simulink model "Copy_2_of_trial_with_intermediate_tanks"  (R2024b)
settings: Solver=ode15s  StartTime=0.0  StopTime=T_sim  FixedStep=1e-6  MaxStep=1e-6  RelTol=1e-6
InitFcn:
  | param = struct();
  | 
  | % Fluid properties
  | param.rho = 870;
  | 
  | % Pressure Rails
  | param.P_H = 7e6;
  | param.P_M = 3.5e6;
  | param.P_L = 101325;
  | 
  | % Linear Actuator Chamber
  | param.V1_0 = 100e-6;
  | param.Acap = pi*(0.5*2.54)^2*1e-4;
  | 
  | % Intermediary volumes
  | param.V3_0 = 25e-6;
  | param.V4_0 = 25e-6;
  | 
  | % Fluid
  | param.beta = 1.8e9;
  | param.air = 0.05;
  | 
  | % Valve
  | param.max_Avt = 0.5*0.25*pi*(20e-3)^2;
  | param.Cd = 0.6;
  | 
  | % Valve Dynamics
  | param.wn = 50*2*pi;
  | param.zeta = 1;
  | 
  | % Hydraulic Pump/Motor
  | param.J_hyd = 3000e-7;
  | param.D = 0.8e-6;    % In cc/rev
  | 
  | % Electric Motor/Generator
  | param.J_elec = 3060e-7;
  | param.Kt = 109e-3;
settings Model: Creator=ibrah408  LastModifiedBy=user
settings SolverCC: MaxConsecutiveZCs=10000
settings RTWCC: GPUComputeCapability=3.5

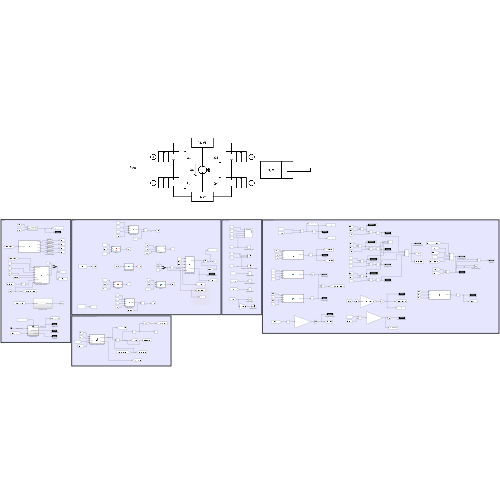
[thumbnail: Simulink's stored preview of the top-level diagram]
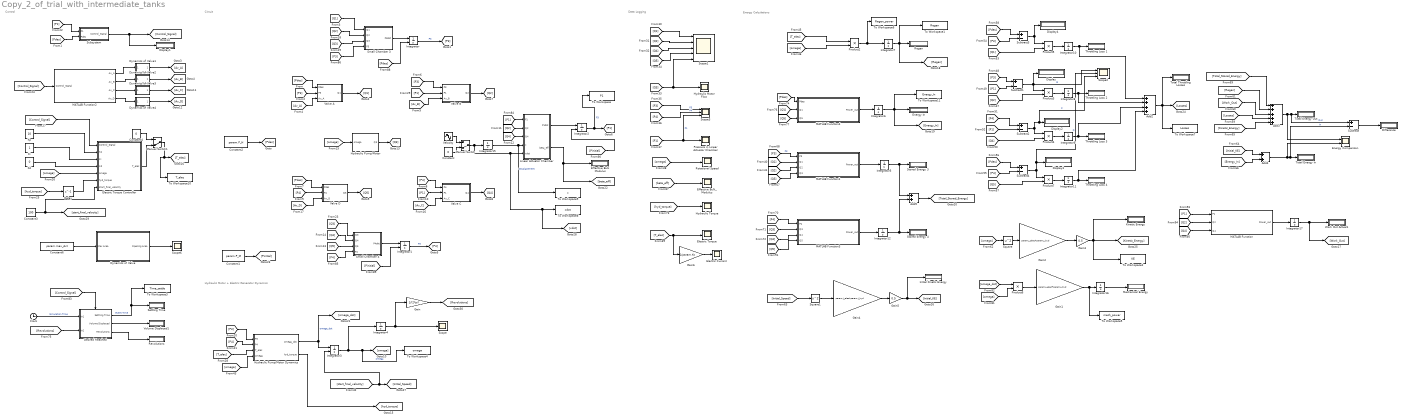
== system Copy_2_of_trial_with_intermediate_tanks ==
  note: Energy Calculations
  note: Data Logging
  note: Hydraulic Motor + Electric Generator Dynamics
  note: Circuit
  note: Control
  Add2 : Sum  Inputs=++++
  Add3 : Sum  Inputs=+++++
  Add4 : Sum
  Add5 : Sum
  Clock : Clock
  Constant : Constant  Value=0
  Constant1 : Constant  Value=param.P_M
  Constant2 : Constant  Value=param.P_H
  Constant3 : Constant  Value=100
  Constant4 : Constant  Value=0
  Constant6 : Constant  Value=param.max_Avt
  Delay : Delay  DelayLength=1
  Desired Reached : Subsystem  TreatAsAtomicUnit=on
  Difference : Display
  Display{,1..4} (5 alike) : Display
  Dynamics of Valve : Subsystem
  Dynamics of Valve1 : Subsystem
  Dynamics of Valve2 : Subsystem
  Dynamics of Valve3 : Subsystem
  Dynamics of Valve4 : Subsystem
  Effective Bulk Modulus : Display
  Effective Bulk_Modulus : Scope
  Electric Current : Scope
  Electric Torque : Scope
  Electric Torque Controller : MATLAB Function  TreatAsAtomicUnit=on
  Energy Comparison : Scope  NumInputPorts=2
  Energy In : Display
  Gain : Gain  Gain=1/(2*pi)
  Gain1 : Gain  Gain=param.J_elec+param.J_hyd
  Gain2 : Gain  Gain=param.J_elec+param.J_hyd
  Gain3 : Gain  Gain=0.5
  Gain4 : Gain  Gain=param.J_elec+param.J_hyd
  Gain5 : Gain  Gain=0.5
  Gain6 : Gain  Gain=1/param.Kt
  Hydraulic Motor Flow : Scope
  Hydraulic Pump/Motor : MATLAB Function  TreatAsAtomicUnit=on
  Hydraulic Pump/Motor Dynamics : MATLAB Function  TreatAsAtomicUnit=on
  Hydraulic Torque : Scope
  Initial Kinetic Energy : Display
  Integrator : Integrator  InitialConditionSource=external  InitialCondition=param.P_M
  Integrator1 : Integrator  InitialConditionSource=external  InitialCondition=param.P_M
  Integrator{4..12,15..17} (12 alike) : Integrator
  Integrator2 : Integrator  InitialConditionSource=external  InitialCondition=param.P_M
  Integrator3 : Integrator  InitialConditionSource=external
  Kd : Constant  Value=0
  Ki : Constant
  Kinetic Energy : Display
  Kp : Constant  Value=10
  Linear Actuator Chamber : MATLAB Function  TreatAsAtomicUnit=on
  MATLAB Function : MATLAB Function  TreatAsAtomicUnit=on
  MATLAB Function1 : MATLAB Function  TreatAsAtomicUnit=on
  MATLAB Function2 : MATLAB Function  TreatAsAtomicUnit=on
  MATLAB Function3 : MATLAB Function  TreatAsAtomicUnit=on
  MATLAB Function4 : MATLAB Function  TreatAsAtomicUnit=on
  Manual Switch : ManualSwitch  CurrentSetting=0
  Manual Switch1 : ManualSwitch  CurrentSetting=0
  Mechanical Energy : Display
  Pressure in Linear Actuator Chamber : Scope
  Product{2..7} (6 alike) : Product
  Regen : Display
  Revolutions : Display
  Rotational Speed : Scope
  Scope : Scope
  Scope1 : Scope  NumInputPorts=5
  Scope2 : Scope  NumInputPorts=3
  Scope3 : Scope  NumInputPorts=3
  Scope6 : Scope
  Settling Time : Display
  Small Chamber 3 : MATLAB Function  TreatAsAtomicUnit=on
  Small Chamber 4 : MATLAB Function  TreatAsAtomicUnit=on
  Square : Math  Operator=square
  Square1 : Math  Operator=square
  Stored Energy 3 : Display
  Stored Energy 4 : Display
  Subsystem : Subsystem
  Subtract{,1..4} (5 alike) : Sum  Inputs=+-
  Throttling Loss {1..4} (4 alike) : Display
  To Workspace : ToWorkspace  VariableName=P1  SaveFormat=Timeseries  SampleTime=-1
  To Workspace1 : ToWorkspace  VariableName=Regen  SaveFormat=Timeseries  SampleTime=-1
  To Workspace10 : ToWorkspace  VariableName=T_elec  SaveFormat=Timeseries  SampleTime=-1
  To Workspace11 : ToWorkspace  VariableName=Energy_In  SaveFormat=Timeseries  SampleTime=-1
  To Workspace2 : ToWorkspace  VariableName=KE  SaveFormat=Timeseries  SampleTime=-1
  To Workspace3 : ToWorkspace  VariableName=Time_settle  SaveFormat=Timeseries  SampleTime=-1
  To Workspace4 : ToWorkspace  VariableName=omega  SaveFormat=Timeseries  SampleTime=-1
  To Workspace5 : ToWorkspace  VariableName=mech_power  SaveFormat=Timeseries  SampleTime=-1
  To Workspace6 : ToWorkspace  VariableName=Regen_power  SaveFormat=Timeseries  SampleTime=-1
  To Workspace7 : ToWorkspace  VariableName=Losses  SaveFormat=Timeseries  SampleTime=-1
  To Workspace8 : ToWorkspace  VariableName=xdot  SaveFormat=Timeseries  SampleTime=-1
  To Workspace9 : ToWorkspace  VariableName=x  SaveFormat=Timeseries  SampleTime=-1
  Total Energy In : Display
  Total Energy Out : Display
  Total Throttling Losses : Display
  Valve A : MATLAB Function  TreatAsAtomicUnit=on
  Valve B : MATLAB Function  TreatAsAtomicUnit=on
  Valve C : MATLAB Function  TreatAsAtomicUnit=on
  Valve D : MATLAB Function  TreatAsAtomicUnit=on
  Velocity : Sin  Amplitude=1e-2  Frequency=(2*pi)/0.2  Phase=pi/2  SampleTime=0
  Volume Displaced1 : Display
  Work Out Actual1 : Display
  wires:
  [Pdes] -> Valve A/1(Pdes)
  Small Chamber 3/1(P3dot) -> Integrator/1
  [Pdes] -> Integrator/2
  Constant2/1 -> [Pdes]
  [Pdes] -> Subsystem/2(Pdes)
  Integrator/1 -> [P3]  "P3"
  [P3] -> Valve A/2(P3)
  Valve A/1(Q1) -> [Q1]
  [Q1] -> Small Chamber 3/1(Q1)
  [Av_A] -> Valve A/3(Av_A)
  [Av_B] -> Valve B/3(Av_B)
  [P3] -> Valve B/1(P3)
  [Pdes] -> Valve D/1(Pdes)
  Small Chamber 4/1(P4dot) -> Integrator1/1
  [Pinitial] -> Integrator1/2
  Integrator1/1 -> [P4]  "P3"
  [P4] -> Valve C/1(P4)
  [P4] -> Valve D/2(P4)
  Linear Actuator Chamber/1(P1dot) -> Integrator2/1
  [Pinitial] -> Integrator2/2
  Integrator2/1 -> To Workspace/1, [P1]  "P3"
  [P1] -> Valve C/2(P1)
  Valve B/1(Q2) -> [Q2]
  [Q2] -> Linear Actuator Chamber/2(Q2)
  Valve C/1(Q4) -> [Q4]
  [Q4] -> Linear Actuator Chamber/3(Q4)
  Valve D/1(Q5) -> [Q5]
  [Q5] -> Small Chamber 4/3(Q5)
  [Q4] -> Small Chamber 4/2(Q4)
  Hydraulic Pump/Motor Dynamics/1(omega_dot) -> [omega_dot], Integrator3/1  "omega_dot"
  Integrator3/1 -> Integrator4/1, To Workspace4/1, [omega]  "omega"
  [omega] -> Hydraulic Pump/Motor/1(omega)
  [Av_C] -> Valve C/3(Av_C)
  [Av_D] -> Valve D/3(Av_D)
  [Q2] -> Small Chamber 3/2(Q2)
  Hydraulic Pump/Motor/1(Q3) -> [Q3]
  [Q3] -> Small Chamber 3/3(Q3)
  [P3] -> Hydraulic Pump/Motor Dynamics/1(P3)
  [P4] -> Hydraulic Pump/Motor Dynamics/2(P4)
  [P1] -> Subsystem/1(P1)
  [Q3] -> Small Chamber 4/1(Q3)
  Subsystem/1(Control_Signal) -> [Control_Signal], Display1/1
  [Control_Signal] -> MATLAB Function2/1(Control_Signal)
  Integrator4/1 -> Scope/1, Gain/1
  Gain/1 -> [Revolutions]
  Hydraulic Pump/Motor Dynamics/2(hyd_torque) -> [hyd_torque]
  [hyd_torque] -> Delay/1
  Delay/1 -> Electric Torque Controller/6(hyd_torque)
  [omega] -> Electric Torque Controller/5(omega)
  [Control_Signal] -> Electric Torque Controller/1(Control_Signal)
  [P1] -> Valve B/2(P1)
  [Q1] -> Scope1/1
  [Q2] -> Scope1/2
  [Q4] -> Scope1/3
  [Q5] -> Scope1/4
  [Q3] -> Scope1/5, Hydraulic Motor Flow/1
  [P3] -> Scope3/1  "P3"
  [P4] -> Scope3/2  "P4"
  [P1] -> Scope3/3, Pressure in Linear Actuator Chamber/1  "P1"
  [omega] -> Rotational Speed/1
  Integrator6/1 -> To Workspace11/1, [Energy_In], Energy In/1
  [T_elec] -> Product2/1
  [omega] -> Product2/2
  Product2/1 -> To Workspace6/1, Integrator7/1
  Integrator7/1 -> To Workspace1/1, [Regen], Regen/1
  Constant6/1 -> Dynamics of Valve/1(Max Area)
  Dynamics of Valve/1(Opening Area) -> Scope6/1
  MATLAB Function2/1(Av_A) -> Dynamics of Valve1/1(Max Area)
  Dynamics of Valve1/1(Opening Area) -> [Av_A]
  MATLAB Function2/2(Av_B) -> Dynamics of Valve2/1(Max Area)
  Dynamics of Valve2/1(Opening Area) -> [Av_B]
  MATLAB Function2/3(Av_C) -> Dynamics of Valve3/1(Max Area)
  Dynamics of Valve3/1(Opening Area) -> [Av_C]
  MATLAB Function2/4(Av_D) -> Dynamics of Valve4/1(Max Area)
  Dynamics of Valve4/1(Opening Area) -> [Av_D]
  Product4/1 -> Integrator9/1
  [Q2] -> Product3/2
  [P4] -> Subtract2/1
  Integrator11/1 -> Add2/4, Throttling Loss 4/1
  [P4] -> Subtract4/2
  [Pdes] -> Subtract4/1
  [P1] -> Subtract2/2
  Product7/1 -> Integrator11/1
  Integrator9/1 -> Add2/3, Throttling Loss 3/1
  Subtract3/1 -> Display4/1, Product5/1
  Product3/1 -> Integrator8/1
  [Pdes] -> Subtract3/1
  Add2/1 -> Total Throttling Losses/1, To Workspace7/1, [Losses]
  Subtract1/1 -> Scope2/1, Product3/1, Display/1  "B"
  Product5/1 -> Integrator10/1
  [P3] -> Subtract1/1
  Integrator8/1 -> Add2/2, Throttling Loss 2/1
  [P1] -> Subtract1/2
  [Q5] -> Product7/2
  Integrator10/1 -> Add2/1, Throttling Loss 1/1
  [P3] -> Subtract3/2
  Subtract4/1 -> Product7/1, Scope2/2, Display3/1  "D"
  [Q4] -> Product4/2
  Subtract2/1 -> Product4/1, Scope2/3, Display2/1  "C"
  [Q1] -> Product5/2
  [Regen] -> Add3/2
  [Work_Out] -> Add3/3
  [Losses] -> Add3/4
  Gain3/1 -> To Workspace2/1, [Kinetic_Energy], Kinetic Energy/1
  [omega] -> Square/1
  Square/1 -> Gain2/1
  Gain2/1 -> Gain3/1
  [Initial_Speed] -> Square1/1
  Gain4/1 -> Gain5/1
  Square1/1 -> Gain4/1
  Gain5/1 -> Initial Kinetic Energy/1, [Initial_KE]
  [Kinetic_Energy] -> Add3/5
  [Initial_KE] -> Add4/1
  [Energy_In] -> Add4/2
  Add4/1 -> Energy Comparison/2, Subtract/2, Total Energy In/1  "In"
  Add3/1 -> Energy Comparison/1, Subtract/1, Total Energy Out/1  "Out"
  Add5/1 -> [Total_Stored_Energy]
  [Total_Stored_Energy] -> Add3/1
  Integrator15/1 -> To Workspace9/1, Linear Actuator Chamber/4(x)  "Displacement"
  Velocity/1 -> Manual Switch/1
  Manual Switch/1 -> Integrator15/1, [xdot], To Workspace8/1, Linear Actuator Chamber/5(xdot)
  Constant/1 -> Manual Switch/2
  Product6/1 -> Gain1/1
  [omega] -> Product6/2
  Integrator16/1 -> Mechanical Energy/1
  [omega_dot] -> Product6/1
  Gain1/1 -> To Workspace5/1, Integrator16/1
  [Control_Signal] -> Desired Reached/Trigger
  Clock/1 -> Desired Reached/1(In1)  "Simulation Time"
  Desired Reached/1(Settling Time) -> Settling Time/1, To Workspace3/1  "Event Time"
  Linear Actuator Chamber/2(beta_eff) -> [beta_eff], Effective Bulk Modulus/1
  [P1] -> Linear Actuator Chamber/1(P1)
  [P4] -> Small Chamber 4/4(P4)
  [P3] -> Small Chamber 3/4(P3)
  [beta_eff] -> Effective Bulk_Modulus/1
  Constant1/1 -> [Pinitial]
  [Q4] -> MATLAB Function/3(Q4)
  [Q2] -> MATLAB Function/2(Q2)
  [P1] -> MATLAB Function/1(P1)
  MATLAB Function/1(Power_out) -> Integrator17/1
  Integrator17/1 -> Work Out Actual1/1, [Work_Out]
  [Q1] -> MATLAB Function1/2(Q1)
  [Q2] -> MATLAB Function1/3(Q2)
  [Q3] -> MATLAB Function1/4(Q3)
  [P3] -> MATLAB Function1/1(P3)  "P3"
  MATLAB Function1/1(Power_out) -> Integrator5/1
  Integrator5/1 -> Add5/1, Stored Energy 3/1
  MATLAB Function3/1(Power_out) -> Integrator12/1
  Integrator12/1 -> Add5/2, Stored Energy 4/1
  [P4] -> MATLAB Function3/1(P4)
  [Q3] -> MATLAB Function3/2(Q3)
  [Q4] -> MATLAB Function3/3(Q4)
  [Q5] -> MATLAB Function3/4(Q5)
  Subtract/1 -> Difference/1
  [hyd_torque] -> Hydraulic Torque/1
  [Revolutions] -> Desired Reached/2(In2)
  Desired Reached/2(Volume Displaced) -> Volume Displaced1/1
  Desired Reached/3(Revolutions) -> Revolutions/1
  [Pdes] -> MATLAB Function4/1(Pdes)
  [Q1] -> MATLAB Function4/2(Q1)
  [Q5] -> MATLAB Function4/3(Q5)
  MATLAB Function4/1(Power_out) -> Integrator6/1
  [T_elec] -> Electric Torque/1, Gain6/1
  Gain6/1 -> Electric Current/1
  Constant3/1 -> Electric Torque Controller/7(start_final_velocity), [start_final_velocity]
  [start_final_velocity] -> [Initial_Speed], Integrator3/2
  [T_elec] -> Hydraulic Pump/Motor Dynamics/3(T_elec)
  Constant4/1 -> Manual Switch1/1
  Electric Torque Controller/1(T_elec) -> Manual Switch1/2
  Manual Switch1/1 -> To Workspace10/1, [T_elec]
  Kp/1 -> Electric Torque Controller/2(Kp)
  Ki/1 -> Electric Torque Controller/3(Ki)
  Kd/1 -> Electric Torque Controller/4(Kd)
  [omega] -> Hydraulic Pump/Motor Dynamics/4(omega)

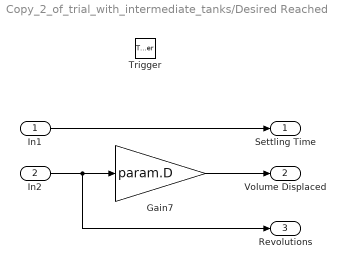
== system Copy_2_of_trial_with_intermediate_tanks/Desired Reached ==
  In1 : Inport
  In2 : Inport  Port=2
  Trigger : TriggerPort  VariantControl=(inherit)
  Gain7 : Gain  Gain=param.D
  Settling Time : Outport
  Volume Displaced : Outport  Port=2
  Revolutions : Outport  Port=3
  wires:
  In1/1 -> Settling Time/1
  Gain7/1 -> Volume Displaced/1
  In2/1 -> Revolutions/1, Gain7/1

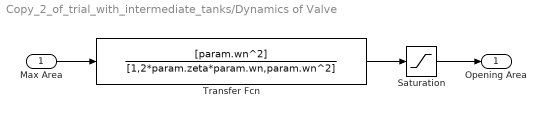
== system Copy_2_of_trial_with_intermediate_tanks/Dynamics of Valve ==
  Max Area : Inport
  Saturation : Saturate  UpperLimit=param.max_Avt  LowerLimit=0
  Transfer Fcn : TransferFcn  Numerator=[param.wn^2]  Denominator=[1,2*param.zeta*param.wn,param.wn^2]
  Opening Area : Outport
  wires:
  Transfer Fcn/1 -> Saturation/1
  Saturation/1 -> Opening Area/1
  Max Area/1 -> Transfer Fcn/1

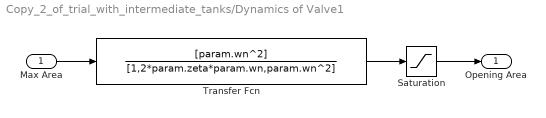
== system Copy_2_of_trial_with_intermediate_tanks/Dynamics of Valve1 ==
  Max Area : Inport
  Saturation : Saturate  UpperLimit=param.max_Avt  LowerLimit=0
  Transfer Fcn : TransferFcn  Numerator=[param.wn^2]  Denominator=[1,2*param.zeta*param.wn,param.wn^2]
  Opening Area : Outport
  wires:
  Max Area/1 -> Transfer Fcn/1
  Saturation/1 -> Opening Area/1
  Transfer Fcn/1 -> Saturation/1

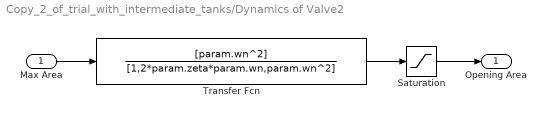
== system Copy_2_of_trial_with_intermediate_tanks/Dynamics of Valve2 ==
  Max Area : Inport
  Saturation : Saturate  UpperLimit=param.max_Avt  LowerLimit=0
  Transfer Fcn : TransferFcn  Numerator=[param.wn^2]  Denominator=[1,2*param.zeta*param.wn,param.wn^2]
  Opening Area : Outport
  wires:
  Transfer Fcn/1 -> Saturation/1
  Saturation/1 -> Opening Area/1
  Max Area/1 -> Transfer Fcn/1

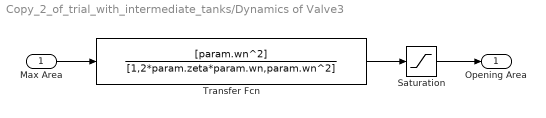
== system Copy_2_of_trial_with_intermediate_tanks/Dynamics of Valve3 ==
  Max Area : Inport
  Saturation : Saturate  UpperLimit=param.max_Avt  LowerLimit=0
  Transfer Fcn : TransferFcn  Numerator=[param.wn^2]  Denominator=[1,2*param.zeta*param.wn,param.wn^2]
  Opening Area : Outport
  wires:
  Max Area/1 -> Transfer Fcn/1
  Saturation/1 -> Opening Area/1
  Transfer Fcn/1 -> Saturation/1

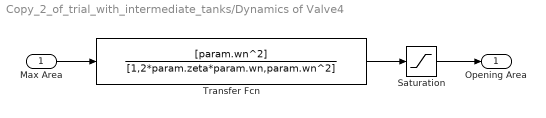
== system Copy_2_of_trial_with_intermediate_tanks/Dynamics of Valve4 ==
  Max Area : Inport
  Saturation : Saturate  UpperLimit=param.max_Avt  LowerLimit=0
  Transfer Fcn : TransferFcn  Numerator=[param.wn^2]  Denominator=[1,2*param.zeta*param.wn,param.wn^2]
  Opening Area : Outport
  wires:
  Transfer Fcn/1 -> Saturation/1
  Saturation/1 -> Opening Area/1
  Max Area/1 -> Transfer Fcn/1

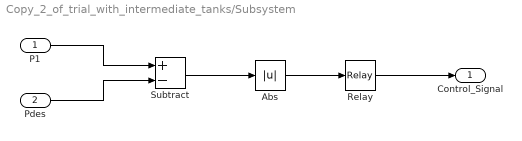
== system Copy_2_of_trial_with_intermediate_tanks/Subsystem ==
  P1 : Inport
  Pdes : Inport  Port=2
  Abs : Abs  SaturateOnIntegerOverflow=off
  Relay : Relay  OnSwitchValue=1e6  OffSwitchValue=1e4  OnOutputValue=0  OffOutputValue=1
  Subtract : Sum  Inputs=+-
  Control_Signal : Outport
  wires:
  P1/1 -> Subtract/1
  Pdes/1 -> Subtract/2
  Subtract/1 -> Abs/1
  Abs/1 -> Relay/1
  Relay/1 -> Control_Signal/1

== matlab function Copy_2_of_trial_with_intermediate_tanks/Hydraulic Pump//Motor ==
  data: omega input; Q3 output; param parameter
function Q3 = fcn(omega, param)

VolEff = 1;
Q3 = VolEff*(param.D/(2*pi))*omega;

== matlab function Copy_2_of_trial_with_intermediate_tanks/Hydraulic Pump//Motor Dynamics ==
  data: P3 input; omega_dot output; P4 input; T_elec input; omega input; param parameter; hyd_torque output
function [omega_dot, hyd_torque] = fcn(P3,P4,T_elec,omega,param)

% 1st term for motoring case, 2nd term for pumping case
MechEff = 1;
dP = P3-P4;
hyd_torque = (omega*dP > 0)*(param.D/(2*pi))*(dP)*MechEff +...
     (omega*dP < 0)*(param.D/(2*pi))*(dP)/MechEff;

% hyd_torque = (param.D/(2*pi))*(P3-P4);
omega_dot = (1/(param.J_elec+param.J_hyd))*(hyd_torque-T_elec);

== matlab function Copy_2_of_trial_with_intermediate_tanks/Electric Torque Controller ==
  data: Control_Signal input; Kp input; Ki input; Kd input; omega input; hyd_torque input; T_elec output; start_final_velocity input
function T_elec  = fcn(Control_Signal, Kp, Ki, Kd, omega, hyd_torque, start_final_velocity)


omega_error_sum_1 = 0;
omega_error_sum_2 = 0;

if Control_Signal == 1 

    if omega < start_final_velocity
        omega_error = -start_final_velocity + omega;

        omega_error_sum_1 = omega_error_sum_1 + omega_error;
        
        T_elec = Kp*omega_error + Ki*omega_error_sum_1;
        % T_elec = hyd_torque;
    else
        T_elec = 1;
    end

else

    if omega >= 120
        omega_error = -120 + omega;

        omega_error_sum_2 = omega_error_sum_2 + omega_error;

        T_elec = Kp*omega_error + Ki*omega_error_sum_2;
        % T_elec = hyd_torque;
    else
        T_elec = -1;
    end

end

== matlab function Copy_2_of_trial_with_intermediate_tanks/MATLAB Function1 ==
  data: P3 input; Q1 input; Q2 input; Q3 input; Power_out output; param parameter
function Power_out = fcn(P3, Q1, Q2, Q3, param)

gamma = 1.4; % Adiabatic process
Pt = param.P_L;

Pg = P3-Pt;   % Gauge pressure
r = P3/Pt;    % Pressure ratio
e = exp(Pg/param.beta);
rv = (1/e+param.air*r^(-1/gamma))/(1+param.air);      %Volume ratio

El=param.beta*(e-(1+Pg/param.beta))+Pt*(e-1);           %Energy in liquid
Eg=P3/(gamma-1).*(1-r.^(1/gamma-1));          %Energy in gas
E=(El./e+param.air*Eg.*r.^(-1/gamma))./(1./e+param.air*r.^(-1/gamma));    %Energy in mixture
W = E-(1./rv-1)*Pt;  %Compressibility (volumetric) energy density

Power_out = (Q1-Q2-Q3)*(W+Pg);

== matlab function Copy_2_of_trial_with_intermediate_tanks/MATLAB Function3 ==
  data: P4 input; Q3 input; Q4 input; Q5 input; Power_out output; param parameter
function Power_out = fcn(P4, Q3, Q4, Q5, param)

gamma = 1.4; % Adiabatic process
Pt = param.P_L;

Pg = P4-Pt;   % Gauge pressure
r = P4/Pt;    % Pressure ratio
e = exp(Pg/param.beta);
rv = (1/e+param.air*r^(-1/gamma))/(1+param.air);      %Volume ratio

El=param.beta*(e-(1+Pg/param.beta))+Pt*(e-1);           %Energy in liquid
Eg=P4/(gamma-1).*(1-r.^(1/gamma-1));          %Energy in gas
E=(El./e+param.air*Eg.*r.^(-1/gamma))./(1./e+param.air*r.^(-1/gamma));    %Energy in mixture
W = E-(1./rv-1)*Pt;  %Compressibility (volumetric) energy density

Power_out = (Q3+Q5-Q4)*(W+Pg);

== matlab function Copy_2_of_trial_with_intermediate_tanks/MATLAB Function4 ==
  data: Pdes input; Q1 input; Q5 input; Power_out output; param parameter
function Power_out = fcn(Pdes, Q1, Q5, param)

gamma = 1.4; % Adiabatic process
Pt = param.P_L;

Pg = Pdes-Pt;   % Gauge pressure
r = Pdes/Pt;    % Pressure ratio
e = exp(Pg/param.beta);
rv = (1/e+param.air*r^(-1/gamma))/(1+param.air);      %Volume ratio

El=param.beta*(e-(1+Pg/param.beta))+Pt*(e-1);           %Energy in liquid
Eg=Pdes/(gamma-1).*(1-r.^(1/gamma-1));          %Energy in gas
E=(El./e+param.air*Eg.*r.^(-1/gamma))./(1./e+param.air*r.^(-1/gamma));    %Energy in mixture
W = E-(1./rv-1)*Pt;  %Compressibility (volumetric) energy density

Power_out = (Q1+Q5)*(W+Pg);

== matlab function Copy_2_of_trial_with_intermediate_tanks/MATLAB Function ==
  data: P1 input; Q2 input; Power_out output; Q4 input; param parameter
function Power_out = fcn(P1, Q2, Q4, param)

gamma = 1.4; % Adiabatic process
Pt = param.P_L;

Pg = P1-Pt;   % Gauge pressure
r = P1/Pt;    % Pressure ratio
e = exp(Pg/param.beta);
rv = (1/e+param.air*r^(-1/gamma))/(1+param.air);      %Volume ratio

El=param.beta*(e-(1+Pg/param.beta))+Pt*(e-1);           %Energy in liquid
Eg=P1/(gamma-1).*(1-r.^(1/gamma-1));          %Energy in gas
E=(El./e+param.air*Eg.*r.^(-1/gamma))./(1./e+param.air*r.^(-1/gamma));    %Energy in mixture
W = E-(1./rv-1)*Pt;  %Compressibility (volumetric) energy density

Power_out = (Q2+Q4)*(W+Pg);

== matlab function Copy_2_of_trial_with_intermediate_tanks/Small Chamber 3 ==
  data: P3dot output; Q1 input; Q2 input; Q3 input; P3 input; param parameter
function P3dot = fcn(Q1, Q2, Q3, P3, param)

gamma = 1.4; % Adiabatic process
Pt = param.P_L;

Pg = P3-Pt;   % Gauge pressure
r = P3/Pt;    % Pressure ratio
e = exp(Pg/param.beta);
rv = (1/e+param.air*r^(-1/gamma))/(1+param.air);      %Volume ratio

% Note: beta_mix as calculated by Hans Barkei
beta_eff = rv*(1+param.air)/(1/(e*param.beta)+param.air/(gamma*Pt*r^(1/gamma+1)));

P3dot = (beta_eff/(param.V3_0))*(Q1-Q2-Q3);

== matlab function Copy_2_of_trial_with_intermediate_tanks/Valve A ==
  data: Pdes input; Q1 output; P3 input; Av_A input; param parameter
function Q1 = fcn(Pdes, P3, Av_A, param)

delP = Pdes - P3;
Q1 = param.Cd*Av_A*sqrt(2/param.rho)*sqrt(abs(delP))*sign(delP);

== matlab function Copy_2_of_trial_with_intermediate_tanks/MATLAB Function2 ==
  data: Control_Signal input; Av_A output; param parameter; Av_B output; Av_C output; Av_D output
function [Av_A, Av_B, Av_C, Av_D] = fcn(Control_Signal, param)

if Control_Signal==1
    
    % Phase 2
    Av_A = param.max_Avt;
    Av_B = param.max_Avt;
    Av_C = 0;
    Av_D = param.max_Avt;

else

    % Phase 1
    Av_A = param.max_Avt;
    Av_B = 0;
    Av_C = param.max_Avt;
    Av_D = 0;

end

== matlab function Copy_2_of_trial_with_intermediate_tanks/Valve B ==
  data: Q2 output; P3 input; P1 input; Av_B input; param parameter
function Q2 = fcn(P3, P1, Av_B, param)

delP = P3 - P1;
Q2 = param.Cd*Av_B*sqrt(2/param.rho)*sqrt(abs(delP))*sign(delP);

== matlab function Copy_2_of_trial_with_intermediate_tanks/Valve D ==
  data: Pdes input; Q5 output; P4 input; Av_D input; param parameter
function Q5 = fcn(Pdes, P4, Av_D, param)

delP = Pdes - P4;
Q5 = param.Cd*Av_D*sqrt(2/param.rho)*sqrt(abs(delP))*sign(delP);

== matlab function Copy_2_of_trial_with_intermediate_tanks/Valve C ==
  data: Q4 output; P4 input; P1 input; Av_C input; param parameter
function Q4 = fcn(P4, P1, Av_C, param)

delP = P4 - P1;
Q4 = param.Cd*Av_C*sqrt(2/param.rho)*sqrt(abs(delP))*sign(delP);

== matlab function Copy_2_of_trial_with_intermediate_tanks/Small Chamber 4 ==
  data: Q3 input; P4dot output; Q4 input; Q5 input; P4 input; param parameter
function P4dot = fcn(Q3, Q4, Q5, P4, param)

gamma = 1.4; % Adiabatic process
Pt = param.P_L;

Pg = P4-Pt;   % Gauge pressure
r = P4/Pt;    % Pressure ratio
e = exp(Pg/param.beta);
rv = (1/e+param.air*r^(-1/gamma))/(1+param.air);      %Volume ratio

% Note: beta_mix as calculated by Hans Barkei
beta_eff = rv*(1+param.air)/(1/(e*param.beta)+param.air/(gamma*Pt*r^(1/gamma+1)));

P4dot = (beta_eff/(param.V4_0))*(Q5+Q3-Q4);

== matlab function Copy_2_of_trial_with_intermediate_tanks/Linear Actuator Chamber ==
  data: P1 input; Q2 input; P1dot output; Q4 input; x input; xdot input; param parameter; beta_eff output
function [P1dot, beta_eff] = fcn(P1,Q2,Q4,x, xdot, param)

gamma = 1.4; % Adiabatic process
Pt = param.P_L;

Pg = P1-Pt;   % Gauge pressure
r = P1/Pt;    % Pressure ratio
e = exp(Pg/param.beta);
rv = (1/e+param.air*r^(-1/gamma))/(1+param.air);      %Volume ratio

% Note: beta_mix as calculated by Hans Barkei
beta_eff = rv*(1+param.air)/(1/(e*param.beta)+param.air/(gamma*Pt*r^(1/gamma+1)));

P1dot = (beta_eff/(param.V1_0+param.Acap*x))*(Q2+Q4-param.Acap*xdot);
